simulink model "simulink_model_integrator"  (R2020b)
settings: Solver=VariableStepAuto  StartTime=0.0  StopTime=10.0  RelTol=1e-3
settings Model: Creator=oj  LastModifiedBy=ydlonari
settings SFSimCC: CustomCodeUndefinedFunction=UseInterfaceOnly

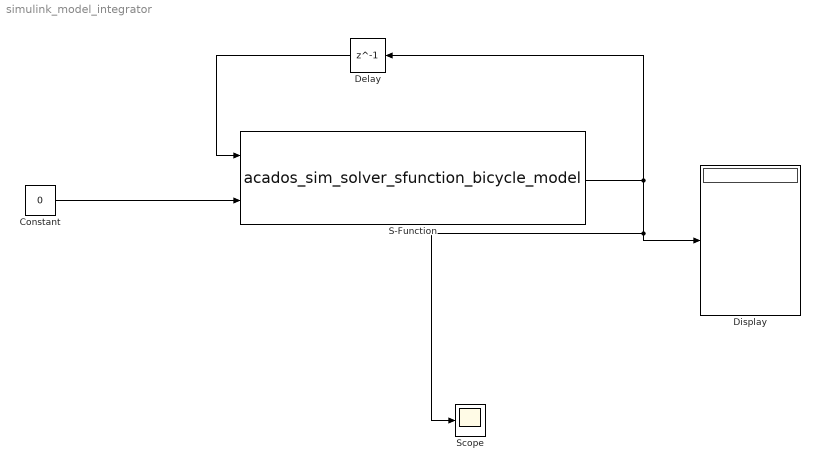
== system simulink_model_integrator ==
  Constant : Constant  Value=0
  Delay : Delay  DelayLength=1  InitialCondition=[0 pi+1 0 0]  SampleTime=1/20
  Display : Display
  S-Function : S-Function  FunctionName=acados_sim_solver_sfunction_bicycle_model  SFunctionDeploymentMode=off  EnableBusSupport=off
  Scope : Scope
  wires:
  Constant/1 -> S-Function/2
  Delay/1 -> S-Function/1
  S-Function/1 -> Scope/1, Display/1, Delay/1
